simulink model "UnityCommunicationTemplate"  (R2019b)
settings: Solver=FixedStepDiscrete  StartTime=0.0  StopTime=inf  FixedStep=1/100  RelTol=1e-3
libraries: xpcutilitieslib x2, xpcrtudplib x2
settings Model: EnablePacing=on  Creator=Aljaz  LastModifiedBy=Aljaz

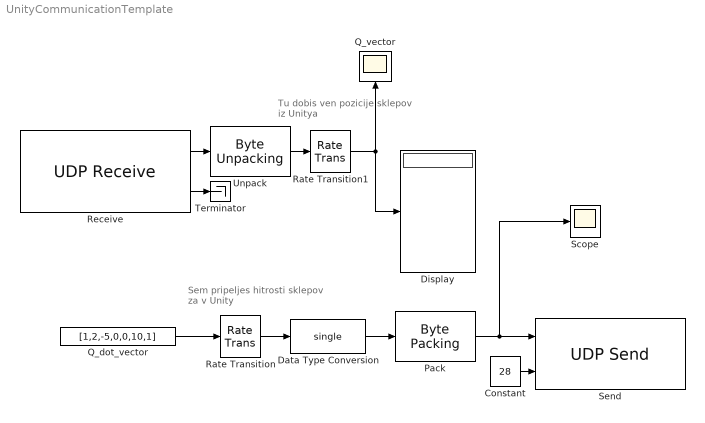
== system UnityCommunicationTemplate ==
  note: Sem pripeljes hitrosti sklepov za v Unity
  note: Tu dobis ven pozicije sklepov iz Unitya
  Constant : Constant  Value=28
  Data Type Conversion : DataTypeConversion  OutDataTypeStr=single
  Display : Display
  Pack : xpcutilitieslib/Byte Packing   MaskPackedDataType=uint8  MaskUnpackedDataTypes={'single'}  MaskAlignment=1
  Q_dot_vector : Constant  Value=[1,2,-5,0,0,10,1]
  Q_vector : Scope
  Rate Transition : RateTransition  InitialCondition=[0 0 0 0 0 0 0]
  Rate Transition1 : RateTransition
  Receive : xpcrtudplib/UDP Receive  ipAddressVal=Use host-target connection  localPort=25106  rcvWidth=7*4  rcvFmAny=off  fmAddress=127.0.0.1  rcvMulticast=off  multicastAddress={}  maxUDPQueue=8  sampleTime=0.01
      settings: SourceProductName=Simulink Real-Time
  Scope : Scope
  Send : xpcrtudplib/UDP Send  ipAddressVal=Use host-target connection  localPort=-1  toAddress=127.0.0.1  toPort=25008  sampleTime=0.01
      settings: SourceProductName=Simulink Real-Time  SourceProductBaseCode=XP
  Terminator : Terminator
  Unpack : xpcutilitieslib/Byte Unpacking   MaskUnpackedDataTypes={'single'}  MaskUnpackedDataSizes={[7]}  MaskAlignment=1
      settings: SourceProductName=Simulink Real-Time  SourceProductBaseCode=XP
  wires:
  Unpack/1 -> Rate Transition1/1
  Rate Transition/1 -> Data Type Conversion/1
  Q_dot_vector/1 -> Rate Transition/1
  Receive/1 -> Unpack/1
  Data Type Conversion/1 -> Pack/1
  Receive/2 -> Terminator/1
  Rate Transition1/1 -> Display/1, Q_vector/1
  Pack/1 -> Scope/1, Send/1
  Constant/1 -> Send/2
